simulink model "celcius_to_fahrenheit"  (R2020b)
settings: Solver=VariableStepAuto  StartTime=0.0  StopTime=10.0  RelTol=1e-3
libraries: simulink x1
settings Model: Creator=Milind  LastModifiedBy=Milind

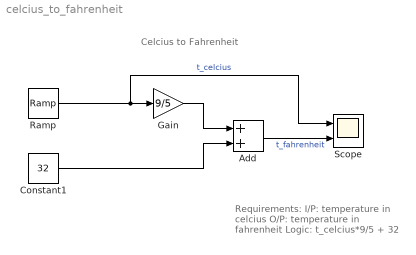
== system celcius_to_fahrenheit ==
  note: Celcius to Fahrenheit
  note: Requirements:
      | I/P: temperature in celcius
      | O/P: temperature in fahrenheit
      | Logic: t_celcius*9/5 + 32
  Add : Sum
  Constant1 : Constant  Value=32
  Gain : Gain  Gain=9/5
  Ramp : simulink/Sources/Ramp  slope=1  start=0  InitialOutput=0
  Scope : Scope  NumInputPorts=2
  wires:
  Ramp/1 -> Scope/1, Gain/1  "t_celcius"
  Gain/1 -> Add/1
  Constant1/1 -> Add/2
  Add/1 -> Scope/2  "t_fahrenheit"
